simulink model "FourRigidBar3D"  (R2025b)
settings: Solver=VariableStepAuto  StartTime=0.0  StopTime=10.0  RelTol=1e-3
undefined symbols (not defined in the file): I2_G, I4_G, InvDyn, l2, l4, m2, m4, pass, sig4, ureal, uss
libraries: RCTblocks x138
(part 1 of 2)
settings Model: Creator=d.alazard  LastModifiedBy=andre
settings SolverCC: AlgebraicLoopSolver=TrustRegion
settings DebuggingCC: AlgebraicLoopMsg=none  UnconnectedInputMsg=warning  UnconnectedOutputMsg=warning  UnconnectedLineMsg=warning
settings ModelReferenceCC: EnableRefExpFcnMdlSchedulingChecks=on
settings RTWCC: GPUComputeCapability=3.5  DLArmComputeVersion=19.05

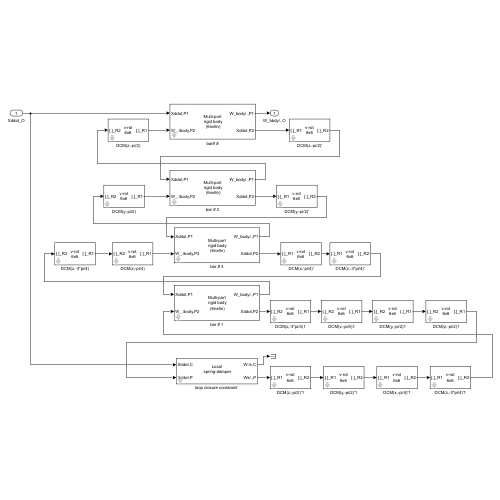
[thumbnail: Simulink's stored preview of the top-level diagram]
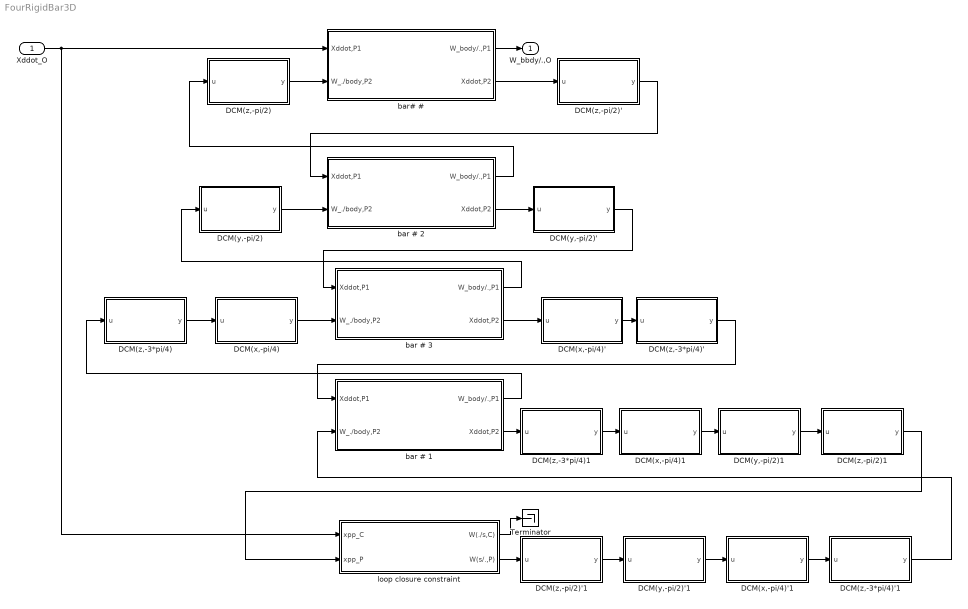
== system FourRigidBar3D ==
  Xddot_O : Inport
  DCM(x,-pi/4) : Subsystem  mask(6x6 rotation matrix (around a given axis)){ra=[1;0;0], theta=-pi/4, transp=off}
      mask prompts: ra "Rotation axis (3x1 vector)"; theta "Angle (rad)"; transp "Matrix transposed"
      mask help:
      | For 6 d.o.f. body motion (3 translations and 3 rotations), this block Implement the 6x6 rotation matrix (or its transposed) for a given angle around a given axis.
      |
      | Angle  (rad) can be an uncertain parameter declared with "ureal" with mode 'Range'
      | Ex: ureal('NAME',0,'Range',[-pi pi])
      | Then, ULINEARIZE will provide a model involving the block named "tan_NAME_div4".
      mask init:
      | vUrotation3x3
      mask Help: web('Doc6vurotation.html','-browser')
      mask Display:
      | disp('v-rot\n6x6')
      | if transp
      |     port_label('input', 1, '[.]_R1')
      |     port_label('output', 1, '[.]_R2')
      | else
      |     port_label('input', 1, '[.]_R2')
      |     port_label('output', 1, '[.]_R1')
      | end
  DCM(x,-pi/4)' : Subsystem  mask(6x6 rotation matrix (around a given axis)){ra=[1;0;0], theta=-pi/4, transp=on}
      mask prompts: ra "Rotation axis (3x1 vector)"; theta "Angle (rad)"; transp "Matrix transposed"
      mask help:
      | For 6 d.o.f. body motion (3 translations and 3 rotations), this block Implement the 6x6 rotation matrix (or its transposed) for a given angle around a given axis.
      |
      | Angle  (rad) can be an uncertain parameter declared with "ureal" with mode 'Range'
      | Ex: ureal('NAME',0,'Range',[-pi pi])
      | Then, ULINEARIZE will provide a model involving the block named "tan_NAME_div4".
      mask init:
      | vUrotation3x3
      mask Help: web('Doc6vurotation.html','-browser')
      mask Display:
      | disp('v-rot\n6x6')
      | if transp
      |     port_label('input', 1, '[.]_R1')
      |     port_label('output', 1, '[.]_R2')
      | else
      |     port_label('input', 1, '[.]_R2')
      |     port_label('output', 1, '[.]_R1')
      | end
  DCM(x,-pi/4)'1 : Subsystem  mask(6x6 rotation matrix (around a given axis)){ra=[1;0;0], theta=-pi/4, transp=on}
      mask prompts: ra "Rotation axis (3x1 vector)"; theta "Angle (rad)"; transp "Matrix transposed"
      mask help:
      | For 6 d.o.f. body motion (3 translations and 3 rotations), this block Implement the 6x6 rotation matrix (or its transposed) for a given angle around a given axis.
      |
      | Angle  (rad) can be an uncertain parameter declared with "ureal" with mode 'Range'
      | Ex: ureal('NAME',0,'Range',[-pi pi])
      | Then, ULINEARIZE will provide a model involving the block named "tan_NAME_div4".
      mask init:
      | vUrotation3x3
      mask Help: web('Doc6vurotation.html','-browser')
      mask Display:
      | disp('v-rot\n6x6')
      | if transp
      |     port_label('input', 1, '[.]_R1')
      |     port_label('output', 1, '[.]_R2')
      | else
      |     port_label('input', 1, '[.]_R2')
      |     port_label('output', 1, '[.]_R1')
      | end
  DCM(x,-pi/4)1 : Subsystem  mask(6x6 rotation matrix (around a given axis)){ra=[1;0;0], theta=-pi/4, transp=off}
      mask prompts: ra "Rotation axis (3x1 vector)"; theta "Angle (rad)"; transp "Matrix transposed"
      mask help:
      | For 6 d.o.f. body motion (3 translations and 3 rotations), this block Implement the 6x6 rotation matrix (or its transposed) for a given angle around a given axis.
      |
      | Angle  (rad) can be an uncertain parameter declared with "ureal" with mode 'Range'
      | Ex: ureal('NAME',0,'Range',[-pi pi])
      | Then, ULINEARIZE will provide a model involving the block named "tan_NAME_div4".
      mask init:
      | vUrotation3x3
      mask Help: web('Doc6vurotation.html','-browser')
      mask Display:
      | disp('v-rot\n6x6')
      | if transp
      |     port_label('input', 1, '[.]_R1')
      |     port_label('output', 1, '[.]_R2')
      | else
      |     port_label('input', 1, '[.]_R2')
      |     port_label('output', 1, '[.]_R1')
      | end
  DCM(y,-pi/2) : Subsystem  mask(6x6 rotation matrix (around a given axis)){ra=[0;1;0], theta=-pi/2, transp=off}
      mask prompts: ra "Rotation axis (3x1 vector)"; theta "Angle (rad)"; transp "Matrix transposed"
      mask help:
      | For 6 d.o.f. body motion (3 translations and 3 rotations), this block Implement the 6x6 rotation matrix (or its transposed) for a given angle around a given axis.
      |
      | Angle  (rad) can be an uncertain parameter declared with "ureal" with mode 'Range'
      | Ex: ureal('NAME',0,'Range',[-pi pi])
      | Then, ULINEARIZE will provide a model involving the block named "tan_NAME_div4".
      mask init:
      | vUrotation3x3
      mask Help: web('Doc6vurotation.html','-browser')
      mask Display:
      | disp('v-rot\n6x6')
      | if transp
      |     port_label('input', 1, '[.]_R1')
      |     port_label('output', 1, '[.]_R2')
      | else
      |     port_label('input', 1, '[.]_R2')
      |     port_label('output', 1, '[.]_R1')
      | end
  DCM(y,-pi/2)' : Subsystem  mask(6x6 rotation matrix (around a given axis)){ra=[0;1;0], theta=-pi/2, transp=on}
      mask prompts: ra "Rotation axis (3x1 vector)"; theta "Angle (rad)"; transp "Matrix transposed"
      mask help:
      | For 6 d.o.f. body motion (3 translations and 3 rotations), this block Implement the 6x6 rotation matrix (or its transposed) for a given angle around a given axis.
      |
      | Angle  (rad) can be an uncertain parameter declared with "ureal" with mode 'Range'
      | Ex: ureal('NAME',0,'Range',[-pi pi])
      | Then, ULINEARIZE will provide a model involving the block named "tan_NAME_div4".
      mask init:
      | vUrotation3x3
      mask Help: web('Doc6vurotation.html','-browser')
      mask Display:
      | disp('v-rot\n6x6')
      | if transp
      |     port_label('input', 1, '[.]_R1')
      |     port_label('output', 1, '[.]_R2')
      | else
      |     port_label('input', 1, '[.]_R2')
      |     port_label('output', 1, '[.]_R1')
      | end
  DCM(y,-pi/2)'1 : Subsystem  mask(6x6 rotation matrix (around a given axis)){ra=[0;1;0], theta=-pi/2, transp=on}
      mask prompts: ra "Rotation axis (3x1 vector)"; theta "Angle (rad)"; transp "Matrix transposed"
      mask help:
      | For 6 d.o.f. body motion (3 translations and 3 rotations), this block Implement the 6x6 rotation matrix (or its transposed) for a given angle around a given axis.
      |
      | Angle  (rad) can be an uncertain parameter declared with "ureal" with mode 'Range'
      | Ex: ureal('NAME',0,'Range',[-pi pi])
      | Then, ULINEARIZE will provide a model involving the block named "tan_NAME_div4".
      mask init:
      | vUrotation3x3
      mask Help: web('Doc6vurotation.html','-browser')
      mask Display:
      | disp('v-rot\n6x6')
      | if transp
      |     port_label('input', 1, '[.]_R1')
      |     port_label('output', 1, '[.]_R2')
      | else
      |     port_label('input', 1, '[.]_R2')
      |     port_label('output', 1, '[.]_R1')
      | end
  DCM(y,-pi/2)1 : Subsystem  mask(6x6 rotation matrix (around a given axis)){ra=[0;1;0], theta=-pi/2, transp=off}
      mask prompts: ra "Rotation axis (3x1 vector)"; theta "Angle (rad)"; transp "Matrix transposed"
      mask help:
      | For 6 d.o.f. body motion (3 translations and 3 rotations), this block Implement the 6x6 rotation matrix (or its transposed) for a given angle around a given axis.
      |
      | Angle  (rad) can be an uncertain parameter declared with "ureal" with mode 'Range'
      | Ex: ureal('NAME',0,'Range',[-pi pi])
      | Then, ULINEARIZE will provide a model involving the block named "tan_NAME_div4".
      mask init:
      | vUrotation3x3
      mask Help: web('Doc6vurotation.html','-browser')
      mask Display:
      | disp('v-rot\n6x6')
      | if transp
      |     port_label('input', 1, '[.]_R1')
      |     port_label('output', 1, '[.]_R2')
      | else
      |     port_label('input', 1, '[.]_R2')
      |     port_label('output', 1, '[.]_R1')
      | end
  DCM(z,-3*pi/4) : Subsystem  mask(6x6 rotation matrix (around a given axis)){ra=[0;0;1], theta=-3*pi/4, transp=off}
      mask prompts: ra "Rotation axis (3x1 vector)"; theta "Angle (rad)"; transp "Matrix transposed"
      mask help:
      | For 6 d.o.f. body motion (3 translations and 3 rotations), this block Implement the 6x6 rotation matrix (or its transposed) for a given angle around a given axis.
      |
      | Angle  (rad) can be an uncertain parameter declared with "ureal" with mode 'Range'
      | Ex: ureal('NAME',0,'Range',[-pi pi])
      | Then, ULINEARIZE will provide a model involving the block named "tan_NAME_div4".
      mask init:
      | vUrotation3x3
      mask Help: web('Doc6vurotation.html','-browser')
      mask Display:
      | disp('v-rot\n6x6')
      | if transp
      |     port_label('input', 1, '[.]_R1')
      |     port_label('output', 1, '[.]_R2')
      | else
      |     port_label('input', 1, '[.]_R2')
      |     port_label('output', 1, '[.]_R1')
      | end
  DCM(z,-3*pi/4)' : Subsystem  mask(6x6 rotation matrix (around a given axis)){ra=[0;0;1], theta=-3*pi/4, transp=on}
      mask prompts: ra "Rotation axis (3x1 vector)"; theta "Angle (rad)"; transp "Matrix transposed"
      mask help:
      | For 6 d.o.f. body motion (3 translations and 3 rotations), this block Implement the 6x6 rotation matrix (or its transposed) for a given angle around a given axis.
      |
      | Angle  (rad) can be an uncertain parameter declared with "ureal" with mode 'Range'
      | Ex: ureal('NAME',0,'Range',[-pi pi])
      | Then, ULINEARIZE will provide a model involving the block named "tan_NAME_div4".
      mask init:
      | vUrotation3x3
      mask Help: web('Doc6vurotation.html','-browser')
      mask Display:
      | disp('v-rot\n6x6')
      | if transp
      |     port_label('input', 1, '[.]_R1')
      |     port_label('output', 1, '[.]_R2')
      | else
      |     port_label('input', 1, '[.]_R2')
      |     port_label('output', 1, '[.]_R1')
      | end
  DCM(z,-3*pi/4)'1 : Subsystem  mask(6x6 rotation matrix (around a given axis)){ra=[0;0;1], theta=-3*pi/4, transp=on}
      mask prompts: ra "Rotation axis (3x1 vector)"; theta "Angle (rad)"; transp "Matrix transposed"
      mask help:
      | For 6 d.o.f. body motion (3 translations and 3 rotations), this block Implement the 6x6 rotation matrix (or its transposed) for a given angle around a given axis.
      |
      | Angle  (rad) can be an uncertain parameter declared with "ureal" with mode 'Range'
      | Ex: ureal('NAME',0,'Range',[-pi pi])
      | Then, ULINEARIZE will provide a model involving the block named "tan_NAME_div4".
      mask init:
      | vUrotation3x3
      mask Help: web('Doc6vurotation.html','-browser')
      mask Display:
      | disp('v-rot\n6x6')
      | if transp
      |     port_label('input', 1, '[.]_R1')
      |     port_label('output', 1, '[.]_R2')
      | else
      |     port_label('input', 1, '[.]_R2')
      |     port_label('output', 1, '[.]_R1')
      | end
  DCM(z,-3*pi/4)1 : Subsystem  mask(6x6 rotation matrix (around a given axis)){ra=[0;0;1], theta=-3*pi/4, transp=off}
      mask prompts: ra "Rotation axis (3x1 vector)"; theta "Angle (rad)"; transp "Matrix transposed"
      mask help:
      | For 6 d.o.f. body motion (3 translations and 3 rotations), this block Implement the 6x6 rotation matrix (or its transposed) for a given angle around a given axis.
      |
      | Angle  (rad) can be an uncertain parameter declared with "ureal" with mode 'Range'
      | Ex: ureal('NAME',0,'Range',[-pi pi])
      | Then, ULINEARIZE will provide a model involving the block named "tan_NAME_div4".
      mask init:
      | vUrotation3x3
      mask Help: web('Doc6vurotation.html','-browser')
      mask Display:
      | disp('v-rot\n6x6')
      | if transp
      |     port_label('input', 1, '[.]_R1')
      |     port_label('output', 1, '[.]_R2')
      | else
      |     port_label('input', 1, '[.]_R2')
      |     port_label('output', 1, '[.]_R1')
      | end
  DCM(z,-pi/2) : Subsystem  mask(6x6 rotation matrix (around a given axis)){ra=[0;0;1], theta=-pi/2, transp=off}
      mask prompts: ra "Rotation axis (3x1 vector)"; theta "Angle (rad)"; transp "Matrix transposed"
      mask help:
      | For 6 d.o.f. body motion (3 translations and 3 rotations), this block Implement the 6x6 rotation matrix (or its transposed) for a given angle around a given axis.
      |
      | Angle  (rad) can be an uncertain parameter declared with "ureal" with mode 'Range'
      | Ex: ureal('NAME',0,'Range',[-pi pi])
      | Then, ULINEARIZE will provide a model involving the block named "tan_NAME_div4".
      mask init:
      | vUrotation3x3
      mask Help: web('Doc6vurotation.html','-browser')
      mask Display:
      | disp('v-rot\n6x6')
      | if transp
      |     port_label('input', 1, '[.]_R1')
      |     port_label('output', 1, '[.]_R2')
      | else
      |     port_label('input', 1, '[.]_R2')
      |     port_label('output', 1, '[.]_R1')
      | end
  DCM(z,-pi/2)' : Subsystem  mask(6x6 rotation matrix (around a given axis)){ra=[0;0;1], theta=-pi/2, transp=on}
      mask prompts: ra "Rotation axis (3x1 vector)"; theta "Angle (rad)"; transp "Matrix transposed"
      mask help:
      | For 6 d.o.f. body motion (3 translations and 3 rotations), this block Implement the 6x6 rotation matrix (or its transposed) for a given angle around a given axis.
      |
      | Angle  (rad) can be an uncertain parameter declared with "ureal" with mode 'Range'
      | Ex: ureal('NAME',0,'Range',[-pi pi])
      | Then, ULINEARIZE will provide a model involving the block named "tan_NAME_div4".
      mask init:
      | vUrotation3x3
      mask Help: web('Doc6vurotation.html','-browser')
      mask Display:
      | disp('v-rot\n6x6')
      | if transp
      |     port_label('input', 1, '[.]_R1')
      |     port_label('output', 1, '[.]_R2')
      | else
      |     port_label('input', 1, '[.]_R2')
      |     port_label('output', 1, '[.]_R1')
      | end
  DCM(z,-pi/2)'1 : Subsystem  mask(6x6 rotation matrix (around a given axis)){ra=[0;0;1], theta=-pi/2, transp=on}
      mask prompts: ra "Rotation axis (3x1 vector)"; theta "Angle (rad)"; transp "Matrix transposed"
      mask help:
      | For 6 d.o.f. body motion (3 translations and 3 rotations), this block Implement the 6x6 rotation matrix (or its transposed) for a given angle around a given axis.
      |
      | Angle  (rad) can be an uncertain parameter declared with "ureal" with mode 'Range'
      | Ex: ureal('NAME',0,'Range',[-pi pi])
      | Then, ULINEARIZE will provide a model involving the block named "tan_NAME_div4".
      mask init:
      | vUrotation3x3
      mask Help: web('Doc6vurotation.html','-browser')
      mask Display:
      | disp('v-rot\n6x6')
      | if transp
      |     port_label('input', 1, '[.]_R1')
      |     port_label('output', 1, '[.]_R2')
      | else
      |     port_label('input', 1, '[.]_R2')
      |     port_label('output', 1, '[.]_R1')
      | end
  DCM(z,-pi/2)1 : Subsystem  mask(6x6 rotation matrix (around a given axis)){ra=[0;0;1], theta=-pi/2, transp=off}
      mask prompts: ra "Rotation axis (3x1 vector)"; theta "Angle (rad)"; transp "Matrix transposed"
      mask help:
      | For 6 d.o.f. body motion (3 translations and 3 rotations), this block Implement the 6x6 rotation matrix (or its transposed) for a given angle around a given axis.
      |
      | Angle  (rad) can be an uncertain parameter declared with "ureal" with mode 'Range'
      | Ex: ureal('NAME',0,'Range',[-pi pi])
      | Then, ULINEARIZE will provide a model involving the block named "tan_NAME_div4".
      mask init:
      | vUrotation3x3
      mask Help: web('Doc6vurotation.html','-browser')
      mask Display:
      | disp('v-rot\n6x6')
      | if transp
      |     port_label('input', 1, '[.]_R1')
      |     port_label('output', 1, '[.]_R2')
      | else
      |     port_label('input', 1, '[.]_R2')
      |     port_label('output', 1, '[.]_R1')
      | end
  Terminator : Terminator
  bar # 1 : Subsystem  mask(Multi-port rigid body (6nx6n)){m=m4, Ig=I4_G, OG=[l4/2;0;0], n=2, numinv=1, OP1=[0;0;0], OP2=[l4;0;0], OP3=[ureal('P3_y',1,'percent',10);0;0], OP4=[0;0;0], OP5=[0;0;0]}
      mask prompts: m "Mass (Kg)"; Ig "Inertia (at G, Kg m^2)"; OG "OG (3x1 vector, m)"; n "Number of ports"; numinv "Port to be inverted"; OP1 "OP1 (3x1 vector, m)"; OP2 "OP2 (3x1 vector, m)"; OP3 "OP3 (3x1 vector, m)"; OP4 "OP4 (3x1 vector, m)"; OP5 "OP5 (3x1 vector,m)"
      mask help:
      | 6nx6n dynamic model of a rigid body at n given points (ports) between wrenches applied at the n points (input) and acceleration twists at these points (output).
      |
      | 0: the reference point
      | G: the center of mass
      | Pi (i=1:n): the n given connection points (n<6).
      |
      | All parameters are expressed in the body frame.
      | Each parameter can be an uncertain parameter declared with "ureal"
      |
      | The 6x6 channel associated to one port can be inverted: then the input of this channel is the acceleration twist imposed at this point and the output is the wrench applied by this body.
      mask init:
      | MultiPortRigidBody
      mask Help: web('Docmultiportrigidbody.html','-browser')
      mask TypeOptions n: 1 | 2 | 3 | 4 | 5
      mask TypeOptions numinv: none | 1 | 2 | 3 | 4 | 5
      mask DialogControl ParameterGroupVar Prompt: Main parameters
      mask DialogControl port1 Prompt: Port #1
      mask DialogControl port2 Prompt: #2
      mask DialogControl port3 Prompt: #3
      mask DialogControl port4 Prompt: #4
      mask DialogControl port5 Prompt: #5
      mask Display:
      | disp('Multi-port\n rigid body\n (6nx6n)')
      | if n==1,
      |     if numinv-1==1,
      |         port_label('input', 1,'Xddot,P')
      |         port_label('output',1,'W_body/.,P')
      |     else
      |         port_label('input', 1,'W_./body,P')
      |         port_label('output',1,'Xddot,P')
      |     end
      | else
      |     for ii=1:n
      |         if numinv==ii+1,
      |             port_label('output',ii,['W_body/.,P',num2str(ii)])
      |             port_label('input', ii,['Xddot,P',num2str(ii)])
      |         else
      |             port_label('input', ii,['W_./body,P',num2str(ii)])
      |             port_label('output',ii,['Xddot,P',num2str(ii)])
      |         end
      |     end
      | end
  bar # 2 : Subsystem  mask(Multi-port rigid body (6nx6n)){m=m2, Ig=I2_G, OG=[l2/2;0;0], n=2, numinv=1, OP1=[0;0;0], OP2=[l2;0;0], OP3=[ureal('P3_y',1,'percent',10);0;0], OP4=[0;0;0], OP5=[0;0;0]}
      mask prompts: m "Mass (Kg)"; Ig "Inertia (at G, Kg m^2)"; OG "OG (3x1 vector, m)"; n "Number of ports"; numinv "Port to be inverted"; OP1 "OP1 (3x1 vector, m)"; OP2 "OP2 (3x1 vector, m)"; OP3 "OP3 (3x1 vector, m)"; OP4 "OP4 (3x1 vector, m)"; OP5 "OP5 (3x1 vector,m)"
      mask help:
      | 6nx6n dynamic model of a rigid body at n given points (ports) between wrenches applied at the n points (input) and acceleration twists at these points (output).
      |
      | 0: the reference point
      | G: the center of mass
      | Pi (i=1:n): the n given connection points (n<6).
      |
      | All parameters are expressed in the body frame.
      | Each parameter can be an uncertain parameter declared with "ureal"
      |
      | The 6x6 channel associated to one port can be inverted: then the input of this channel is the acceleration twist imposed at this point and the output is the wrench applied by this body.
      mask init:
      | MultiPortRigidBody
      mask Help: web('Docmultiportrigidbody.html','-browser')
      mask TypeOptions n: 1 | 2 | 3 | 4 | 5
      mask TypeOptions numinv: none | 1 | 2 | 3 | 4 | 5
      mask DialogControl ParameterGroupVar Prompt: Main parameters
      mask DialogControl port1 Prompt: Port #1
      mask DialogControl port2 Prompt: #2
      mask DialogControl port3 Prompt: #3
      mask DialogControl port4 Prompt: #4
      mask DialogControl port5 Prompt: #5
      mask Display:
      | disp('Multi-port\n rigid body\n (6nx6n)')
      | if n==1,
      |     if numinv-1==1,
      |         port_label('input', 1,'Xddot,P')
      |         port_label('output',1,'W_body/.,P')
      |     else
      |         port_label('input', 1,'W_./body,P')
      |         port_label('output',1,'Xddot,P')
      |     end
      | else
      |     for ii=1:n
      |         if numinv==ii+1,
      |             port_label('output',ii,['W_body/.,P',num2str(ii)])
      |             port_label('input', ii,['Xddot,P',num2str(ii)])
      |         else
      |             port_label('input', ii,['W_./body,P',num2str(ii)])
      |             port_label('output',ii,['Xddot,P',num2str(ii)])
      |         end
      |     end
      | end
  bar # 3 : Subsystem  mask(Multi-port rigid body (6nx6n)){m=m2, Ig=I2_G, OG=[l2/2;0;0], n=2, numinv=1, OP1=[0;0;0], OP2=[l2;0;0], OP3=[ureal('P3_y',1,'percent',10);0;0], OP4=[0;0;0], OP5=[0;0;0]}
      mask prompts: m "Mass (Kg)"; Ig "Inertia (at G, Kg m^2)"; OG "OG (3x1 vector, m)"; n "Number of ports"; numinv "Port to be inverted"; OP1 "OP1 (3x1 vector, m)"; OP2 "OP2 (3x1 vector, m)"; OP3 "OP3 (3x1 vector, m)"; OP4 "OP4 (3x1 vector, m)"; OP5 "OP5 (3x1 vector,m)"
      mask help:
      | 6nx6n dynamic model of a rigid body at n given points (ports) between wrenches applied at the n points (input) and acceleration twists at these points (output).
      |
      | 0: the reference point
      | G: the center of mass
      | Pi (i=1:n): the n given connection points (n<6).
      |
      | All parameters are expressed in the body frame.
      | Each parameter can be an uncertain parameter declared with "ureal"
      |
      | The 6x6 channel associated to one port can be inverted: then the input of this channel is the acceleration twist imposed at this point and the output is the wrench applied by this body.
      mask init:
      | MultiPortRigidBody
      mask Help: web('Docmultiportrigidbody.html','-browser')
      mask TypeOptions n: 1 | 2 | 3 | 4 | 5
      mask TypeOptions numinv: none | 1 | 2 | 3 | 4 | 5
      mask DialogControl ParameterGroupVar Prompt: Main parameters
      mask DialogControl port1 Prompt: Port #1
      mask DialogControl port2 Prompt: #2
      mask DialogControl port3 Prompt: #3
      mask DialogControl port4 Prompt: #4
      mask DialogControl port5 Prompt: #5
      mask Display:
      | disp('Multi-port\n rigid body\n (6nx6n)')
      | if n==1,
      |     if numinv-1==1,
      |         port_label('input', 1,'Xddot,P')
      |         port_label('output',1,'W_body/.,P')
      |     else
      |         port_label('input', 1,'W_./body,P')
      |         port_label('output',1,'Xddot,P')
      |     end
      | else
      |     for ii=1:n
      |         if numinv==ii+1,
      |             port_label('output',ii,['W_body/.,P',num2str(ii)])
      |             port_label('input', ii,['Xddot,P',num2str(ii)])
      |         else
      |             port_label('input', ii,['W_./body,P',num2str(ii)])
      |             port_label('output',ii,['Xddot,P',num2str(ii)])
      |         end
      |     end
      | end
  bar# # : Subsystem  mask(Multi-port rigid body (6nx6n)){m=m2, Ig=I2_G, OG=[l2/2;0;0], n=2, numinv=1, OP1=[0;0;0], OP2=[l2;0;0], OP3=[ureal('P3_y',1,'percent',10);0;0], OP4=[0;0;0], OP5=[0;0;0]}
      mask prompts: m "Mass (Kg)"; Ig "Inertia (at G, Kg m^2)"; OG "OG (3x1 vector, m)"; n "Number of ports"; numinv "Port to be inverted"; OP1 "OP1 (3x1 vector, m)"; OP2 "OP2 (3x1 vector, m)"; OP3 "OP3 (3x1 vector, m)"; OP4 "OP4 (3x1 vector, m)"; OP5 "OP5 (3x1 vector,m)"
      mask help:
      | 6nx6n dynamic model of a rigid body at n given points (ports) between wrenches applied at the n points (input) and acceleration twists at these points (output).
      |
      | 0: the reference point
      | G: the center of mass
      | Pi (i=1:n): the n given connection points (n<6).
      |
      | All parameters are expressed in the body frame.
      | Each parameter can be an uncertain parameter declared with "ureal"
      |
      | The 6x6 channel associated to one port can be inverted: then the input of this channel is the acceleration twist imposed at this point and the output is the wrench applied by this body.
      mask init:
      | MultiPortRigidBody
      mask Help: web('Docmultiportrigidbody.html','-browser')
      mask TypeOptions n: 1 | 2 | 3 | 4 | 5
      mask TypeOptions numinv: none | 1 | 2 | 3 | 4 | 5
      mask DialogControl ParameterGroupVar Prompt: Main parameters
      mask DialogControl port1 Prompt: Port #1
      mask DialogControl port2 Prompt: #2
      mask DialogControl port3 Prompt: #3
      mask DialogControl port4 Prompt: #4
      mask DialogControl port5 Prompt: #5
      mask Display:
      | disp('Multi-port\n rigid body\n (6nx6n)')
      | if n==1,
      |     if numinv-1==1,
      |         port_label('input', 1,'Xddot,P')
      |         port_label('output',1,'W_body/.,P')
      |     else
      |         port_label('input', 1,'W_./body,P')
      |         port_label('output',1,'Xddot,P')
      |     end
      | else
      |     for ii=1:n
      |         if numinv==ii+1,
      |             port_label('output',ii,['W_body/.,P',num2str(ii)])
      |             port_label('input', ii,['Xddot,P',num2str(ii)])
      |         else
      |             port_label('input', ii,['W_./body,P',num2str(ii)])
      |             port_label('output',ii,['Xddot,P',num2str(ii)])
      |         end
      |     end
      | end
  "loop closure constraint " : Subsystem  mask(Local stiffness damper){K_O=diag([1 1 1 2 2 2]), D_O=diag([10 10 10 20 20 20]), OP=[0;0;0], OC=[0;0;0]}
      mask prompts: K_O "6x6 stiffness matrix at point O (N/m, Nm/rad)"; D_O "6x6 damping matrix  at point O (Ns/m, Nms/rad)"; OP "OP (3x1 vector (m)"; OC "OC (3x1 vector  (m)"
      mask help:
      | 12x12 TITOP model of a massless spring-damper system between:
      |   * the 2 acceleration twists (inputs)  at the parent port (point P) and the child port (point C).
      |   *  the outside wrench applied to the spring-damper  at point C and the wrench by the spring-damper to outside at point P.
      | The model is expressed In the inherit reference frame.
      |
      | All the parameters can be declared as uncertain parameters (ureal(...)).
      mask init:
      | TAU_OC=kinematic_model([0;0;0],OC);
      | TAU_OP=kinematic_model([0;0;0],OP);
      mask Help: web('Doc_6DOFs_spring_damper.html','-browser')
      mask DialogControl ParameterGroupVar Prompt: Main parameters
      mask Display:
      | disp('Local\n spring-damper\n')
      | 
      | port_label('input', 1,'Xddot,C')
      | port_label('output',1,'W./s,C')
      | port_label('input', 2,'Xddot,P')
      | port_label('output',2,'Ws/.,P')
  W_bbdy/.,O : Outport
  wires:
  Xddot_O/1 -> "loop closure constraint "/1(xpp_C), bar# #/1(Xddot,P1)
  bar# #/2(Xddot,P2) -> DCM(z,-pi/2)'/1(u)
  DCM(z,-pi/2)/1(y) -> bar# #/2(W_./body,P2)
  DCM(z,-pi/2)'/1(y) -> bar # 2/1(Xddot,P1)
  bar # 2/1(W_body/.,P1) -> DCM(z,-pi/2)/1(u)
  bar # 2/2(Xddot,P2) -> DCM(y,-pi/2)'/1(u)
  DCM(y,-pi/2)/1(y) -> bar # 2/2(W_./body,P2)
  DCM(y,-pi/2)'/1(y) -> bar # 3/1(Xddot,P1)
  bar # 3/1(W_body/.,P1) -> DCM(y,-pi/2)/1(u)
  bar # 3/2(Xddot,P2) -> DCM(x,-pi/4)'/1(u)
  DCM(x,-pi/4)/1(y) -> bar # 3/2(W_./body,P2)
  DCM(x,-pi/4)'/1(y) -> DCM(z,-3*pi/4)'/1(u)
  DCM(z,-3*pi/4)/1(y) -> DCM(x,-pi/4)/1(u)
  DCM(z,-3*pi/4)'/1(y) -> bar # 1/1(Xddot,P1)
  bar # 1/1(W_body/.,P1) -> DCM(z,-3*pi/4)/1(u)
  bar # 1/2(Xddot,P2) -> DCM(z,-3*pi/4)1/1(u)
  DCM(z,-3*pi/4)1/1(y) -> DCM(x,-pi/4)1/1(u)
  DCM(x,-pi/4)1/1(y) -> DCM(y,-pi/2)1/1(u)
  DCM(y,-pi/2)1/1(y) -> DCM(z,-pi/2)1/1(u)
  DCM(z,-pi/2)1/1(y) -> "loop closure constraint "/2(xpp_P)
  "loop closure constraint "/2(W(s/.,P)) -> DCM(z,-pi/2)'1/1(u)
  bar# #/1(W_body/.,P1) -> W_bbdy/.,O/1
  DCM(z,-pi/2)'1/1(y) -> DCM(y,-pi/2)'1/1(u)
  DCM(y,-pi/2)'1/1(y) -> DCM(x,-pi/4)'1/1(u)
  DCM(x,-pi/4)'1/1(y) -> DCM(z,-3*pi/4)'1/1(u)
  DCM(z,-3*pi/4)'1/1(y) -> bar # 1/2(W_./body,P2)
  "loop closure constraint "/1(W(./s,C)) -> Terminator/1

== system FourRigidBar3D/DCM(x,-pi//4) ==
  u : Inport  PortDimensions=6
  Demux : Demux  Outputs=[3 3]
  Mux : Mux  Inputs=[3 3]
  Subsystem : Subsystem
  Subsystem1 : Subsystem
  y : Outport  VectorParamsAs1DForOutWhenUnconnected=off
  wires:
  Subsystem1/1(Out1) -> Mux/2
  Subsystem/1(Out1) -> Mux/1
  Demux/2 -> Subsystem1/1(In1)
  Demux/1 -> Subsystem/1(In1)
  u/1 -> Demux/1
  Mux/1 -> y/1

== system FourRigidBar3D/DCM(x,-pi//4)' ==
  u : Inport  PortDimensions=6
  Demux : Demux  Outputs=[3 3]
  Mux : Mux  Inputs=[3 3]
  Subsystem : Subsystem
  Subsystem1 : Subsystem
  y : Outport  VectorParamsAs1DForOutWhenUnconnected=off
  wires:
  Subsystem1/1(Out1) -> Mux/2
  Subsystem/1(Out1) -> Mux/1
  Demux/2 -> Subsystem1/1(In1)
  Demux/1 -> Subsystem/1(In1)
  u/1 -> Demux/1
  Mux/1 -> y/1

== system FourRigidBar3D/DCM(x,-pi//4)'1 ==
  u : Inport  PortDimensions=6
  Demux : Demux  Outputs=[3 3]
  Mux : Mux  Inputs=[3 3]
  Subsystem : Subsystem
  Subsystem1 : Subsystem
  y : Outport  VectorParamsAs1DForOutWhenUnconnected=off
  wires:
  Subsystem1/1(Out1) -> Mux/2
  Subsystem/1(Out1) -> Mux/1
  Demux/2 -> Subsystem1/1(In1)
  Demux/1 -> Subsystem/1(In1)
  u/1 -> Demux/1
  Mux/1 -> y/1

== system FourRigidBar3D/DCM(x,-pi//4)1 ==
  u : Inport  PortDimensions=6
  Demux : Demux  Outputs=[3 3]
  Mux : Mux  Inputs=[3 3]
  Subsystem : Subsystem
  Subsystem1 : Subsystem
  y : Outport  VectorParamsAs1DForOutWhenUnconnected=off
  wires:
  Subsystem1/1(Out1) -> Mux/2
  Subsystem/1(Out1) -> Mux/1
  Demux/2 -> Subsystem1/1(In1)
  Demux/1 -> Subsystem/1(In1)
  u/1 -> Demux/1
  Mux/1 -> y/1

== system FourRigidBar3D/DCM(y,-pi//2) ==
  u : Inport  PortDimensions=6
  Demux : Demux  Outputs=[3 3]
  Mux : Mux  Inputs=[3 3]
  Subsystem : Subsystem
  Subsystem1 : Subsystem
  y : Outport  VectorParamsAs1DForOutWhenUnconnected=off
  wires:
  Subsystem1/1(Out1) -> Mux/2
  Subsystem/1(Out1) -> Mux/1
  Demux/2 -> Subsystem1/1(In1)
  Demux/1 -> Subsystem/1(In1)
  u/1 -> Demux/1
  Mux/1 -> y/1

== system FourRigidBar3D/DCM(y,-pi//2)' ==
  u : Inport  PortDimensions=6
  Demux : Demux  Outputs=[3 3]
  Mux : Mux  Inputs=[3 3]
  Subsystem : Subsystem
  Subsystem1 : Subsystem
  y : Outport  VectorParamsAs1DForOutWhenUnconnected=off
  wires:
  Subsystem1/1(Out1) -> Mux/2
  Subsystem/1(Out1) -> Mux/1
  Demux/2 -> Subsystem1/1(In1)
  Demux/1 -> Subsystem/1(In1)
  u/1 -> Demux/1
  Mux/1 -> y/1

== system FourRigidBar3D/DCM(y,-pi//2)'1 ==
  u : Inport  PortDimensions=6
  Demux : Demux  Outputs=[3 3]
  Mux : Mux  Inputs=[3 3]
  Subsystem : Subsystem
  Subsystem1 : Subsystem
  y : Outport  VectorParamsAs1DForOutWhenUnconnected=off
  wires:
  Subsystem1/1(Out1) -> Mux/2
  Subsystem/1(Out1) -> Mux/1
  Demux/2 -> Subsystem1/1(In1)
  Demux/1 -> Subsystem/1(In1)
  u/1 -> Demux/1
  Mux/1 -> y/1

== system FourRigidBar3D/DCM(y,-pi//2)1 ==
  u : Inport  PortDimensions=6
  Demux : Demux  Outputs=[3 3]
  Mux : Mux  Inputs=[3 3]
  Subsystem : Subsystem
  Subsystem1 : Subsystem
  y : Outport  VectorParamsAs1DForOutWhenUnconnected=off
  wires:
  Subsystem1/1(Out1) -> Mux/2
  Subsystem/1(Out1) -> Mux/1
  Demux/2 -> Subsystem1/1(In1)
  Demux/1 -> Subsystem/1(In1)
  u/1 -> Demux/1
  Mux/1 -> y/1

== system FourRigidBar3D/DCM(z,-3*pi//4) ==
  u : Inport  PortDimensions=6
  Demux : Demux  Outputs=[3 3]
  Mux : Mux  Inputs=[3 3]
  Subsystem : Subsystem
  Subsystem1 : Subsystem
  y : Outport  VectorParamsAs1DForOutWhenUnconnected=off
  wires:
  Subsystem1/1(Out1) -> Mux/2
  Subsystem/1(Out1) -> Mux/1
  Demux/2 -> Subsystem1/1(In1)
  Demux/1 -> Subsystem/1(In1)
  u/1 -> Demux/1
  Mux/1 -> y/1

== system FourRigidBar3D/DCM(z,-3*pi//4)' ==
  u : Inport  PortDimensions=6
  Demux : Demux  Outputs=[3 3]
  Mux : Mux  Inputs=[3 3]
  Subsystem : Subsystem
  Subsystem1 : Subsystem
  y : Outport  VectorParamsAs1DForOutWhenUnconnected=off
  wires:
  Subsystem1/1(Out1) -> Mux/2
  Subsystem/1(Out1) -> Mux/1
  Demux/2 -> Subsystem1/1(In1)
  Demux/1 -> Subsystem/1(In1)
  u/1 -> Demux/1
  Mux/1 -> y/1

== system FourRigidBar3D/DCM(z,-3*pi//4)'1 ==
  u : Inport  PortDimensions=6
  Demux : Demux  Outputs=[3 3]
  Mux : Mux  Inputs=[3 3]
  Subsystem : Subsystem
  Subsystem1 : Subsystem
  y : Outport  VectorParamsAs1DForOutWhenUnconnected=off
  wires:
  Subsystem1/1(Out1) -> Mux/2
  Subsystem/1(Out1) -> Mux/1
  Demux/2 -> Subsystem1/1(In1)
  Demux/1 -> Subsystem/1(In1)
  u/1 -> Demux/1
  Mux/1 -> y/1

== system FourRigidBar3D/DCM(z,-3*pi//4)1 ==
  u : Inport  PortDimensions=6
  Demux : Demux  Outputs=[3 3]
  Mux : Mux  Inputs=[3 3]
  Subsystem : Subsystem
  Subsystem1 : Subsystem
  y : Outport  VectorParamsAs1DForOutWhenUnconnected=off
  wires:
  Subsystem1/1(Out1) -> Mux/2
  Subsystem/1(Out1) -> Mux/1
  Demux/2 -> Subsystem1/1(In1)
  Demux/1 -> Subsystem/1(In1)
  u/1 -> Demux/1
  Mux/1 -> y/1

== system FourRigidBar3D/DCM(z,-pi//2) ==
  u : Inport  PortDimensions=6
  Demux : Demux  Outputs=[3 3]
  Mux : Mux  Inputs=[3 3]
  Subsystem : Subsystem
  Subsystem1 : Subsystem
  y : Outport  VectorParamsAs1DForOutWhenUnconnected=off
  wires:
  Subsystem1/1(Out1) -> Mux/2
  Subsystem/1(Out1) -> Mux/1
  Demux/2 -> Subsystem1/1(In1)
  Demux/1 -> Subsystem/1(In1)
  u/1 -> Demux/1
  Mux/1 -> y/1

== system FourRigidBar3D/DCM(z,-pi//2)' ==
  u : Inport  PortDimensions=6
  Demux : Demux  Outputs=[3 3]
  Mux : Mux  Inputs=[3 3]
  Subsystem : Subsystem
  Subsystem1 : Subsystem
  y : Outport  VectorParamsAs1DForOutWhenUnconnected=off
  wires:
  Subsystem1/1(Out1) -> Mux/2
  Subsystem/1(Out1) -> Mux/1
  Demux/2 -> Subsystem1/1(In1)
  Demux/1 -> Subsystem/1(In1)
  u/1 -> Demux/1
  Mux/1 -> y/1

== system FourRigidBar3D/DCM(z,-pi//2)'1 ==
  u : Inport  PortDimensions=6
  Demux : Demux  Outputs=[3 3]
  Mux : Mux  Inputs=[3 3]
  Subsystem : Subsystem
  Subsystem1 : Subsystem
  y : Outport  VectorParamsAs1DForOutWhenUnconnected=off
  wires:
  Subsystem1/1(Out1) -> Mux/2
  Subsystem/1(Out1) -> Mux/1
  Demux/2 -> Subsystem1/1(In1)
  Demux/1 -> Subsystem/1(In1)
  u/1 -> Demux/1
  Mux/1 -> y/1

== system FourRigidBar3D/DCM(z,-pi//2)1 ==
  u : Inport  PortDimensions=6
  Demux : Demux  Outputs=[3 3]
  Mux : Mux  Inputs=[3 3]
  Subsystem : Subsystem
  Subsystem1 : Subsystem
  y : Outport  VectorParamsAs1DForOutWhenUnconnected=off
  wires:
  Subsystem1/1(Out1) -> Mux/2
  Subsystem/1(Out1) -> Mux/1
  Demux/2 -> Subsystem1/1(In1)
  Demux/1 -> Subsystem/1(In1)
  u/1 -> Demux/1
  Mux/1 -> y/1

== system FourRigidBar3D/bar # 1 ==
  Xddot,P1 : Inport  PortDimensions=6
  W_./body,P2 : Inport  Port=2  PortDimensions=6
  Demux : Demux  Outputs=[6 6]
  Gain : RCTblocks/Uncertain State Space  Tag=USS  USystem=uss(InvDyn)  UValue=[]  X0=[]  uX0=[]
  Mux : Mux  Inputs=[6 6]
  W_body/.,P1 : Outport
  Xddot,P2 : Outport  Port=2
  wires:
  Demux/2 -> Xddot,P2/1
  W_./body,P2/1 -> Mux/2
  Demux/1 -> W_body/.,P1/1
  Xddot,P1/1 -> Mux/1
  Gain/1 -> Demux/1
  Mux/1 -> Gain/1

== system FourRigidBar3D/bar # 2 ==
  Xddot,P1 : Inport  PortDimensions=6
  W_./body,P2 : Inport  Port=2  PortDimensions=6
  Demux : Demux  Outputs=[6 6]
  Gain : RCTblocks/Uncertain State Space  Tag=USS  USystem=uss(InvDyn)  UValue=[]  X0=[]  uX0=[]
  Mux : Mux  Inputs=[6 6]
  W_body/.,P1 : Outport
  Xddot,P2 : Outport  Port=2
  wires:
  Demux/2 -> Xddot,P2/1
  W_./body,P2/1 -> Mux/2
  Demux/1 -> W_body/.,P1/1
  Xddot,P1/1 -> Mux/1
  Gain/1 -> Demux/1
  Mux/1 -> Gain/1

== system FourRigidBar3D/bar # 3 ==
  Xddot,P1 : Inport  PortDimensions=6
  W_./body,P2 : Inport  Port=2  PortDimensions=6
  Demux : Demux  Outputs=[6 6]
  Gain : RCTblocks/Uncertain State Space  Tag=USS  USystem=uss(InvDyn)  UValue=[]  X0=[]  uX0=[]
  Mux : Mux  Inputs=[6 6]
  W_body/.,P1 : Outport
  Xddot,P2 : Outport  Port=2
  wires:
  Mux/1 -> Gain/1
  Gain/1 -> Demux/1
  Xddot,P1/1 -> Mux/1
  Demux/1 -> W_body/.,P1/1
  W_./body,P2/1 -> Mux/2
  Demux/2 -> Xddot,P2/1

== system FourRigidBar3D/bar# # ==
  Xddot,P1 : Inport  PortDimensions=6
  W_./body,P2 : Inport  Port=2  PortDimensions=6
  Demux : Demux  Outputs=[6 6]
  Gain : RCTblocks/Uncertain State Space  Tag=USS  USystem=uss(InvDyn)  UValue=[]  X0=[]  uX0=[]
  Mux : Mux  Inputs=[6 6]
  W_body/.,P1 : Outport
  Xddot,P2 : Outport  Port=2
  wires:
  Mux/1 -> Gain/1
  Gain/1 -> Demux/1
  Xddot,P1/1 -> Mux/1
  Demux/1 -> W_body/.,P1/1
  W_./body,P2/1 -> Mux/2
  Demux/2 -> Xddot,P2/1

== system FourRigidBar3D/loop closure constraint  ==
  xpp_C : Inport  PortDimensions=6
  xpp_P : Inport  Port=2  PortDimensions=6
  Damping Matrix : RCTblocks/Uncertain State Space  Tag=USS  USystem=ss(D_O)  UValue=[]  X0=[]  uX0=[]
  Damping Matrix1 : RCTblocks/Uncertain State Space  Tag=USS  USystem=ss(K_O)  UValue=[]  X0=[]  uX0=[]
  Integrator 1 : Integrator
  Integrator 2 : Integrator
  Kinematic model between O and C : RCTblocks/Uncertain State Space  Tag=USS  USystem=ss(TAU_OC)  UValue=[]  X0=[]  uX0=[]
  Kinematic model between O and C' : RCTblocks/Uncertain State Space  Tag=USS  USystem=ss(TAU_OC')  UValue=[]  X0=[]  uX0=[]
  Kinematic model between O and P : RCTblocks/Uncertain State Space  Tag=USS  USystem=ss(TAU_OP)  UValue=[]  X0=[]  uX0=[]
  Kinematic model between O and P' : RCTblocks/Uncertain State Space  Tag=USS  USystem=ss(TAU_OP')  UValue=[]  X0=[]  uX0=[]
  Sum : Sum  Inputs=|+-
  Sum1 : Sum  Inputs=++|
  W(./s,C) : Outport  VectorParamsAs1DForOutWhenUnconnected=off
  W(s/.,P) : Outport  Port=2  VectorParamsAs1DForOutWhenUnconnected=off
  wires:
  Kinematic model between O and C'/1 -> W(./s,C)/1
  Kinematic model between O and P'/1 -> W(s/.,P)/1
  xpp_P/1 -> Kinematic model between O and P/1
  Integrator 1/1 -> Integrator 2/1, Damping Matrix/1
  xpp_C/1 -> Kinematic model between O and C/1
  Kinematic model between O and C/1 -> Sum/1
  Sum/1 -> Integrator 1/1
  Kinematic model between O and P/1 -> Sum/2
  Damping Matrix/1 -> Sum1/2
  Damping Matrix1/1 -> Sum1/1
  Integrator 2/1 -> Damping Matrix1/1
  Sum1/1 -> Kinematic model between O and C'/1, Kinematic model between O and P'/1

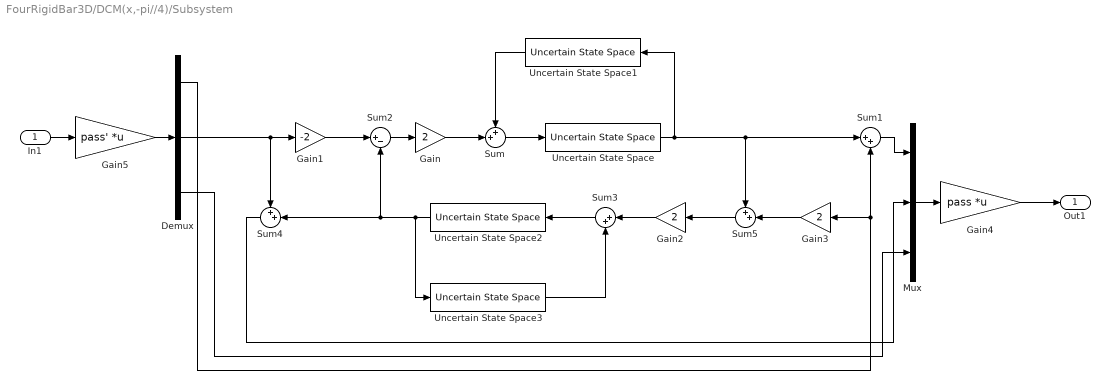
== system FourRigidBar3D/DCM(x,-pi//4)/Subsystem ==
  In1 : Inport
  Demux : Demux  Outputs=3
  Gain : Gain  Gain=2
  Gain1 : Gain  Gain=-2
  Gain2 : Gain  Gain=2
  Gain3 : Gain  Gain=2
  Gain4 : Gain  Gain=pass  Multiplication=Matrix(K*u) (u vector)
  Gain5 : Gain  Gain=pass'  Multiplication=Matrix(K*u) (u vector)
  Mux : Mux  Inputs=3
  Sum : Sum  Inputs=++|
  Sum1 : Sum  Inputs=|++
  Sum2 : Sum  Inputs=|+-
  Sum3 : Sum  Inputs=|++
  Sum4 : Sum  Inputs=++|
  Sum5 : Sum  Inputs=++|
  Uncertain State Space{,1..3} (4 alike) : RCTblocks/Uncertain State Space  Tag=USS  USystem=uss(sig4)  UValue=[]  X0=[]  uX0=[]
  Out1 : Outport  VectorParamsAs1DForOutWhenUnconnected=off
  wires:
  Gain5/1 -> Demux/1
  Gain4/1 -> Out1/1
  Uncertain State Space3/1 -> Sum3/2
  Gain2/1 -> Sum3/1
  In1/1 -> Gain5/1
  Gain/1 -> Sum/2
  Uncertain State Space2/1 -> Uncertain State Space3/1, Sum4/2, Sum2/2
  Demux/1 -> Gain3/1, Sum1/2
  Demux/3 -> Mux/3
  Mux/1 -> Gain4/1
  Sum4/1 -> Mux/2
  Sum3/1 -> Uncertain State Space2/1
  Gain1/1 -> Sum2/1
  Uncertain State Space/1 -> Uncertain State Space1/1, Sum5/1, Sum1/1
  Gain3/1 -> Sum5/2
  Sum/1 -> Uncertain State Space/1
  Demux/2 -> Sum4/1, Gain1/1
  Uncertain State Space1/1 -> Sum/1
  Sum2/1 -> Gain/1
  Sum1/1 -> Mux/1
  Sum5/1 -> Gain2/1

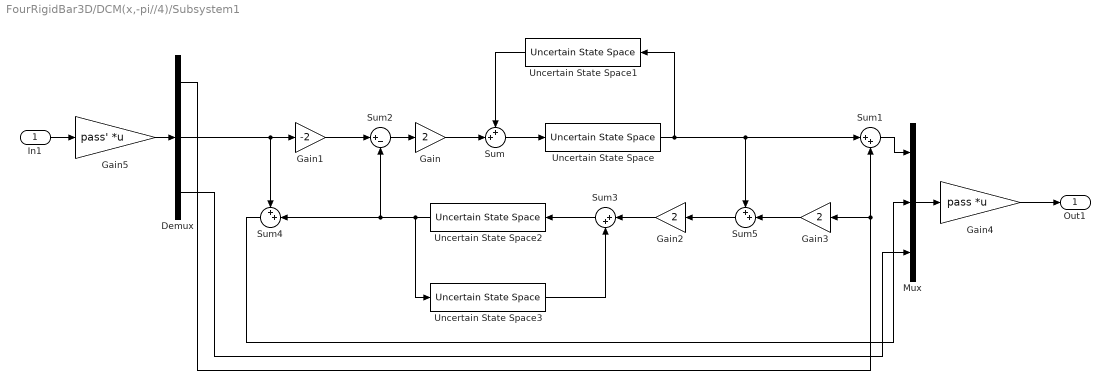
== system FourRigidBar3D/DCM(x,-pi//4)/Subsystem1 ==
  In1 : Inport
  Demux : Demux  Outputs=3
  Gain : Gain  Gain=2
  Gain1 : Gain  Gain=-2
  Gain2 : Gain  Gain=2
  Gain3 : Gain  Gain=2
  Gain4 : Gain  Gain=pass  Multiplication=Matrix(K*u) (u vector)
  Gain5 : Gain  Gain=pass'  Multiplication=Matrix(K*u) (u vector)
  Mux : Mux  Inputs=3
  Sum : Sum  Inputs=++|
  Sum1 : Sum  Inputs=|++
  Sum2 : Sum  Inputs=|+-
  Sum3 : Sum  Inputs=|++
  Sum4 : Sum  Inputs=++|
  Sum5 : Sum  Inputs=++|
  Uncertain State Space{,1..3} (4 alike) : RCTblocks/Uncertain State Space  Tag=USS  USystem=uss(sig4)  UValue=[]  X0=[]  uX0=[]
  Out1 : Outport  VectorParamsAs1DForOutWhenUnconnected=off
  wires:
  Gain5/1 -> Demux/1
  Sum5/1 -> Gain2/1
  Sum1/1 -> Mux/1
  Sum2/1 -> Gain/1
  Uncertain State Space1/1 -> Sum/1
  Demux/2 -> Gain1/1, Sum4/1
  Sum/1 -> Uncertain State Space/1
  Gain3/1 -> Sum5/2
  Uncertain State Space/1 -> Sum1/1, Sum5/1, Uncertain State Space1/1
  Gain1/1 -> Sum2/1
  Sum3/1 -> Uncertain State Space2/1
  Sum4/1 -> Mux/2
  Mux/1 -> Gain4/1
  Demux/3 -> Mux/3
  Demux/1 -> Sum1/2, Gain3/1
  Uncertain State Space2/1 -> Sum2/2, Sum4/2, Uncertain State Space3/1
  Gain/1 -> Sum/2
  In1/1 -> Gain5/1
  Gain2/1 -> Sum3/1
  Uncertain State Space3/1 -> Sum3/2
  Gain4/1 -> Out1/1

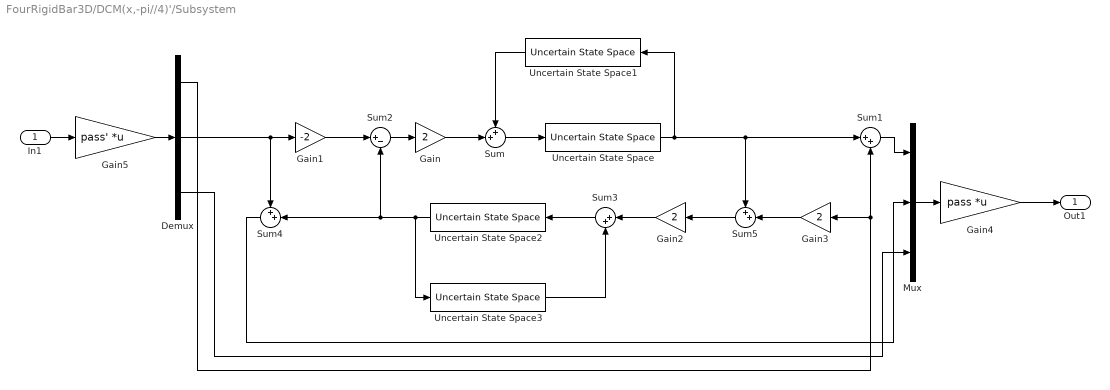
== system FourRigidBar3D/DCM(x,-pi//4)'/Subsystem ==
  In1 : Inport
  Demux : Demux  Outputs=3
  Gain : Gain  Gain=2
  Gain1 : Gain  Gain=-2
  Gain2 : Gain  Gain=2
  Gain3 : Gain  Gain=2
  Gain4 : Gain  Gain=pass  Multiplication=Matrix(K*u) (u vector)
  Gain5 : Gain  Gain=pass'  Multiplication=Matrix(K*u) (u vector)
  Mux : Mux  Inputs=3
  Sum : Sum  Inputs=++|
  Sum1 : Sum  Inputs=|++
  Sum2 : Sum  Inputs=|+-
  Sum3 : Sum  Inputs=|++
  Sum4 : Sum  Inputs=++|
  Sum5 : Sum  Inputs=++|
  Uncertain State Space{,1..3} (4 alike) : RCTblocks/Uncertain State Space  Tag=USS  USystem=uss(sig4)  UValue=[]  X0=[]  uX0=[]
  Out1 : Outport  VectorParamsAs1DForOutWhenUnconnected=off
  wires:
  Gain5/1 -> Demux/1
  Gain4/1 -> Out1/1
  Uncertain State Space3/1 -> Sum3/2
  Gain2/1 -> Sum3/1
  In1/1 -> Gain5/1
  Gain/1 -> Sum/2
  Uncertain State Space2/1 -> Uncertain State Space3/1, Sum4/2, Sum2/2
  Demux/1 -> Gain3/1, Sum1/2
  Demux/3 -> Mux/3
  Mux/1 -> Gain4/1
  Sum4/1 -> Mux/2
  Sum3/1 -> Uncertain State Space2/1
  Gain1/1 -> Sum2/1
  Uncertain State Space/1 -> Uncertain State Space1/1, Sum5/1, Sum1/1
  Gain3/1 -> Sum5/2
  Sum/1 -> Uncertain State Space/1
  Demux/2 -> Sum4/1, Gain1/1
  Uncertain State Space1/1 -> Sum/1
  Sum2/1 -> Gain/1
  Sum1/1 -> Mux/1
  Sum5/1 -> Gain2/1

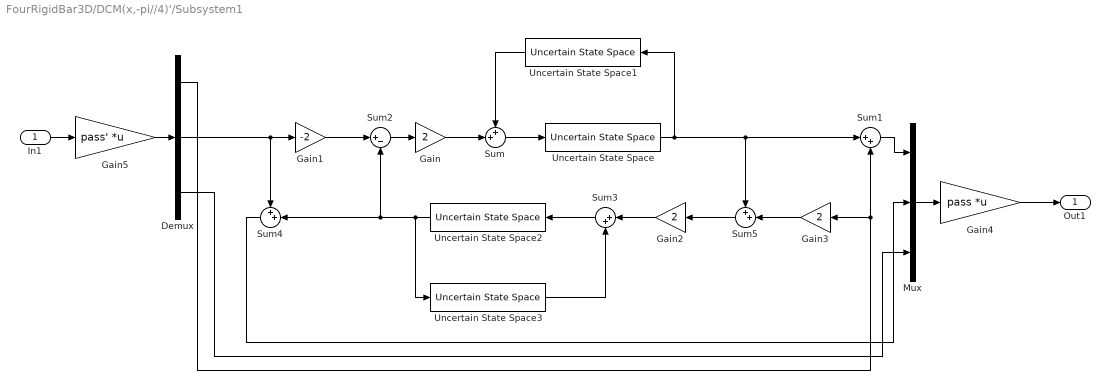
== system FourRigidBar3D/DCM(x,-pi//4)'/Subsystem1 ==
  In1 : Inport
  Demux : Demux  Outputs=3
  Gain : Gain  Gain=2
  Gain1 : Gain  Gain=-2
  Gain2 : Gain  Gain=2
  Gain3 : Gain  Gain=2
  Gain4 : Gain  Gain=pass  Multiplication=Matrix(K*u) (u vector)
  Gain5 : Gain  Gain=pass'  Multiplication=Matrix(K*u) (u vector)
  Mux : Mux  Inputs=3
  Sum : Sum  Inputs=++|
  Sum1 : Sum  Inputs=|++
  Sum2 : Sum  Inputs=|+-
  Sum3 : Sum  Inputs=|++
  Sum4 : Sum  Inputs=++|
  Sum5 : Sum  Inputs=++|
  Uncertain State Space{,1..3} (4 alike) : RCTblocks/Uncertain State Space  Tag=USS  USystem=uss(sig4)  UValue=[]  X0=[]  uX0=[]
  Out1 : Outport  VectorParamsAs1DForOutWhenUnconnected=off
  wires:
  Gain5/1 -> Demux/1
  Sum5/1 -> Gain2/1
  Sum1/1 -> Mux/1
  Sum2/1 -> Gain/1
  Uncertain State Space1/1 -> Sum/1
  Demux/2 -> Gain1/1, Sum4/1
  Sum/1 -> Uncertain State Space/1
  Gain3/1 -> Sum5/2
  Uncertain State Space/1 -> Sum1/1, Sum5/1, Uncertain State Space1/1
  Gain1/1 -> Sum2/1
  Sum3/1 -> Uncertain State Space2/1
  Sum4/1 -> Mux/2
  Mux/1 -> Gain4/1
  Demux/3 -> Mux/3
  Demux/1 -> Sum1/2, Gain3/1
  Uncertain State Space2/1 -> Sum2/2, Sum4/2, Uncertain State Space3/1
  Gain/1 -> Sum/2
  In1/1 -> Gain5/1
  Gain2/1 -> Sum3/1
  Uncertain State Space3/1 -> Sum3/2
  Gain4/1 -> Out1/1

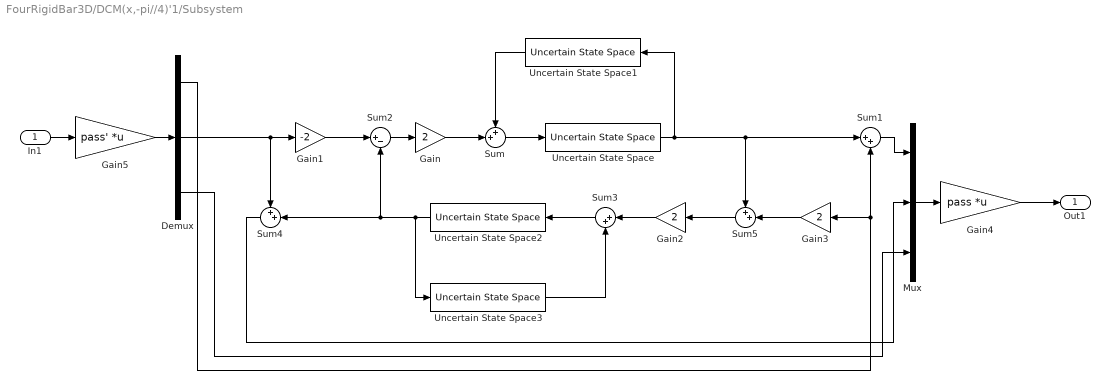
== system FourRigidBar3D/DCM(x,-pi//4)'1/Subsystem ==
  In1 : Inport
  Demux : Demux  Outputs=3
  Gain : Gain  Gain=2
  Gain1 : Gain  Gain=-2
  Gain2 : Gain  Gain=2
  Gain3 : Gain  Gain=2
  Gain4 : Gain  Gain=pass  Multiplication=Matrix(K*u) (u vector)
  Gain5 : Gain  Gain=pass'  Multiplication=Matrix(K*u) (u vector)
  Mux : Mux  Inputs=3
  Sum : Sum  Inputs=++|
  Sum1 : Sum  Inputs=|++
  Sum2 : Sum  Inputs=|+-
  Sum3 : Sum  Inputs=|++
  Sum4 : Sum  Inputs=++|
  Sum5 : Sum  Inputs=++|
  Uncertain State Space{,1..3} (4 alike) : RCTblocks/Uncertain State Space  Tag=USS  USystem=uss(sig4)  UValue=[]  X0=[]  uX0=[]
  Out1 : Outport  VectorParamsAs1DForOutWhenUnconnected=off
  wires:
  Gain5/1 -> Demux/1
  Gain4/1 -> Out1/1
  Uncertain State Space3/1 -> Sum3/2
  Gain2/1 -> Sum3/1
  In1/1 -> Gain5/1
  Gain/1 -> Sum/2
  Uncertain State Space2/1 -> Uncertain State Space3/1, Sum4/2, Sum2/2
  Demux/1 -> Gain3/1, Sum1/2
  Demux/3 -> Mux/3
  Mux/1 -> Gain4/1
  Sum4/1 -> Mux/2
  Sum3/1 -> Uncertain State Space2/1
  Gain1/1 -> Sum2/1
  Uncertain State Space/1 -> Uncertain State Space1/1, Sum5/1, Sum1/1
  Gain3/1 -> Sum5/2
  Sum/1 -> Uncertain State Space/1
  Demux/2 -> Sum4/1, Gain1/1
  Uncertain State Space1/1 -> Sum/1
  Sum2/1 -> Gain/1
  Sum1/1 -> Mux/1
  Sum5/1 -> Gain2/1

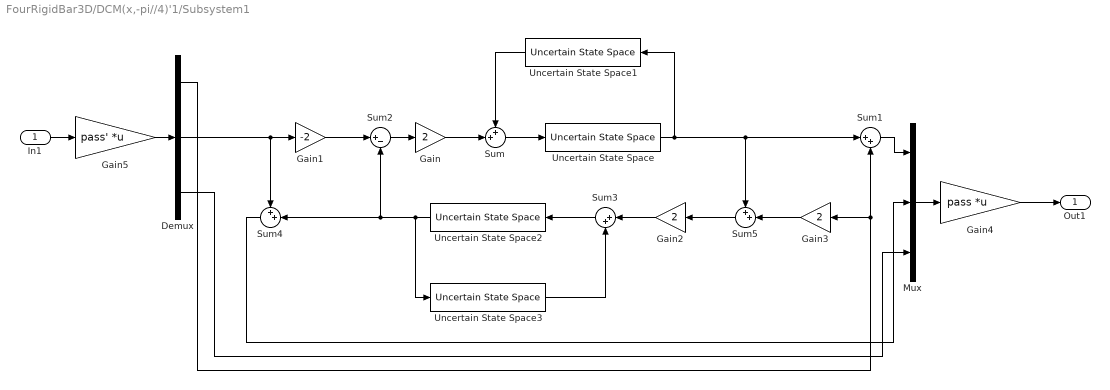
== system FourRigidBar3D/DCM(x,-pi//4)'1/Subsystem1 ==
  In1 : Inport
  Demux : Demux  Outputs=3
  Gain : Gain  Gain=2
  Gain1 : Gain  Gain=-2
  Gain2 : Gain  Gain=2
  Gain3 : Gain  Gain=2
  Gain4 : Gain  Gain=pass  Multiplication=Matrix(K*u) (u vector)
  Gain5 : Gain  Gain=pass'  Multiplication=Matrix(K*u) (u vector)
  Mux : Mux  Inputs=3
  Sum : Sum  Inputs=++|
  Sum1 : Sum  Inputs=|++
  Sum2 : Sum  Inputs=|+-
  Sum3 : Sum  Inputs=|++
  Sum4 : Sum  Inputs=++|
  Sum5 : Sum  Inputs=++|
  Uncertain State Space{,1..3} (4 alike) : RCTblocks/Uncertain State Space  Tag=USS  USystem=uss(sig4)  UValue=[]  X0=[]  uX0=[]
  Out1 : Outport  VectorParamsAs1DForOutWhenUnconnected=off
  wires:
  Gain5/1 -> Demux/1
  Sum5/1 -> Gain2/1
  Sum1/1 -> Mux/1
  Sum2/1 -> Gain/1
  Uncertain State Space1/1 -> Sum/1
  Demux/2 -> Gain1/1, Sum4/1
  Sum/1 -> Uncertain State Space/1
  Gain3/1 -> Sum5/2
  Uncertain State Space/1 -> Sum1/1, Sum5/1, Uncertain State Space1/1
  Gain1/1 -> Sum2/1
  Sum3/1 -> Uncertain State Space2/1
  Sum4/1 -> Mux/2
  Mux/1 -> Gain4/1
  Demux/3 -> Mux/3
  Demux/1 -> Sum1/2, Gain3/1
  Uncertain State Space2/1 -> Sum2/2, Sum4/2, Uncertain State Space3/1
  Gain/1 -> Sum/2
  In1/1 -> Gain5/1
  Gain2/1 -> Sum3/1
  Uncertain State Space3/1 -> Sum3/2
  Gain4/1 -> Out1/1

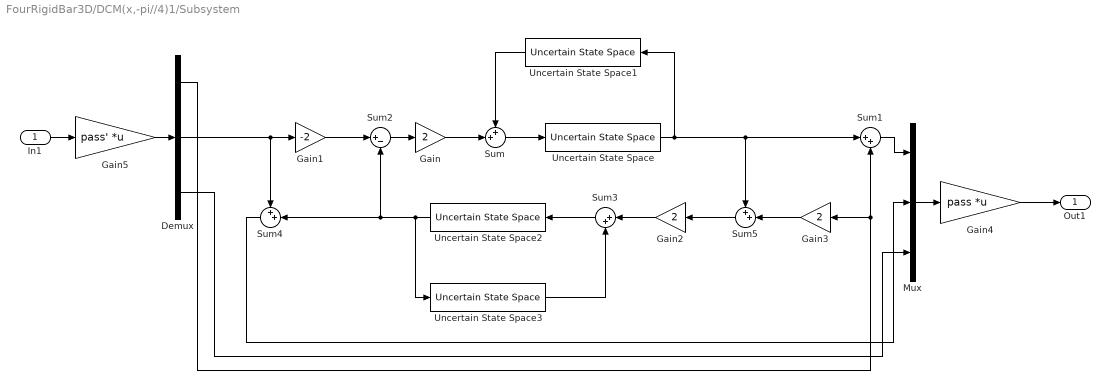
== system FourRigidBar3D/DCM(x,-pi//4)1/Subsystem ==
  In1 : Inport
  Demux : Demux  Outputs=3
  Gain : Gain  Gain=2
  Gain1 : Gain  Gain=-2
  Gain2 : Gain  Gain=2
  Gain3 : Gain  Gain=2
  Gain4 : Gain  Gain=pass  Multiplication=Matrix(K*u) (u vector)
  Gain5 : Gain  Gain=pass'  Multiplication=Matrix(K*u) (u vector)
  Mux : Mux  Inputs=3
  Sum : Sum  Inputs=++|
  Sum1 : Sum  Inputs=|++
  Sum2 : Sum  Inputs=|+-
  Sum3 : Sum  Inputs=|++
  Sum4 : Sum  Inputs=++|
  Sum5 : Sum  Inputs=++|
  Uncertain State Space{,1..3} (4 alike) : RCTblocks/Uncertain State Space  Tag=USS  USystem=uss(sig4)  UValue=[]  X0=[]  uX0=[]
  Out1 : Outport  VectorParamsAs1DForOutWhenUnconnected=off
  wires:
  Gain5/1 -> Demux/1
  Gain4/1 -> Out1/1
  Uncertain State Space3/1 -> Sum3/2
  Gain2/1 -> Sum3/1
  In1/1 -> Gain5/1
  Gain/1 -> Sum/2
  Uncertain State Space2/1 -> Uncertain State Space3/1, Sum4/2, Sum2/2
  Demux/1 -> Gain3/1, Sum1/2
  Demux/3 -> Mux/3
  Mux/1 -> Gain4/1
  Sum4/1 -> Mux/2
  Sum3/1 -> Uncertain State Space2/1
  Gain1/1 -> Sum2/1
  Uncertain State Space/1 -> Uncertain State Space1/1, Sum5/1, Sum1/1
  Gain3/1 -> Sum5/2
  Sum/1 -> Uncertain State Space/1
  Demux/2 -> Sum4/1, Gain1/1
  Uncertain State Space1/1 -> Sum/1
  Sum2/1 -> Gain/1
  Sum1/1 -> Mux/1
  Sum5/1 -> Gain2/1

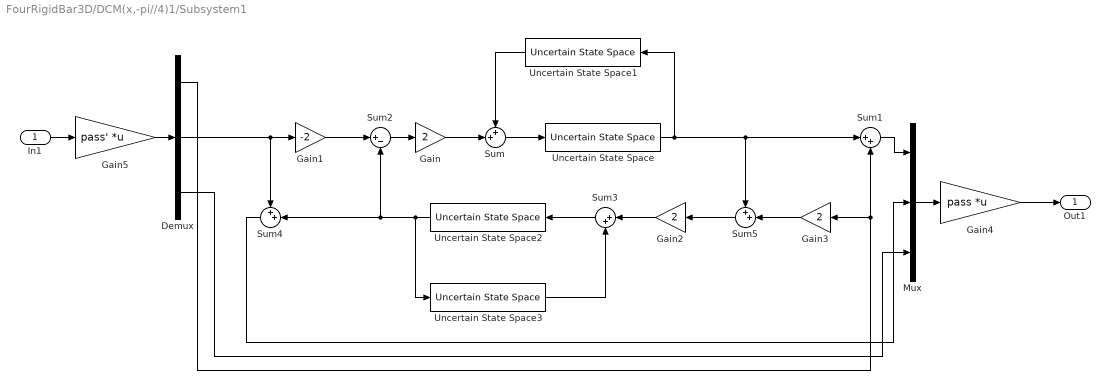
== system FourRigidBar3D/DCM(x,-pi//4)1/Subsystem1 ==
  In1 : Inport
  Demux : Demux  Outputs=3
  Gain : Gain  Gain=2
  Gain1 : Gain  Gain=-2
  Gain2 : Gain  Gain=2
  Gain3 : Gain  Gain=2
  Gain4 : Gain  Gain=pass  Multiplication=Matrix(K*u) (u vector)
  Gain5 : Gain  Gain=pass'  Multiplication=Matrix(K*u) (u vector)
  Mux : Mux  Inputs=3
  Sum : Sum  Inputs=++|
  Sum1 : Sum  Inputs=|++
  Sum2 : Sum  Inputs=|+-
  Sum3 : Sum  Inputs=|++
  Sum4 : Sum  Inputs=++|
  Sum5 : Sum  Inputs=++|
  Uncertain State Space{,1..3} (4 alike) : RCTblocks/Uncertain State Space  Tag=USS  USystem=uss(sig4)  UValue=[]  X0=[]  uX0=[]
  Out1 : Outport  VectorParamsAs1DForOutWhenUnconnected=off
  wires:
  Gain5/1 -> Demux/1
  Sum5/1 -> Gain2/1
  Sum1/1 -> Mux/1
  Sum2/1 -> Gain/1
  Uncertain State Space1/1 -> Sum/1
  Demux/2 -> Gain1/1, Sum4/1
  Sum/1 -> Uncertain State Space/1
  Gain3/1 -> Sum5/2
  Uncertain State Space/1 -> Sum1/1, Sum5/1, Uncertain State Space1/1
  Gain1/1 -> Sum2/1
  Sum3/1 -> Uncertain State Space2/1
  Sum4/1 -> Mux/2
  Mux/1 -> Gain4/1
  Demux/3 -> Mux/3
  Demux/1 -> Sum1/2, Gain3/1
  Uncertain State Space2/1 -> Sum2/2, Sum4/2, Uncertain State Space3/1
  Gain/1 -> Sum/2
  In1/1 -> Gain5/1
  Gain2/1 -> Sum3/1
  Uncertain State Space3/1 -> Sum3/2
  Gain4/1 -> Out1/1

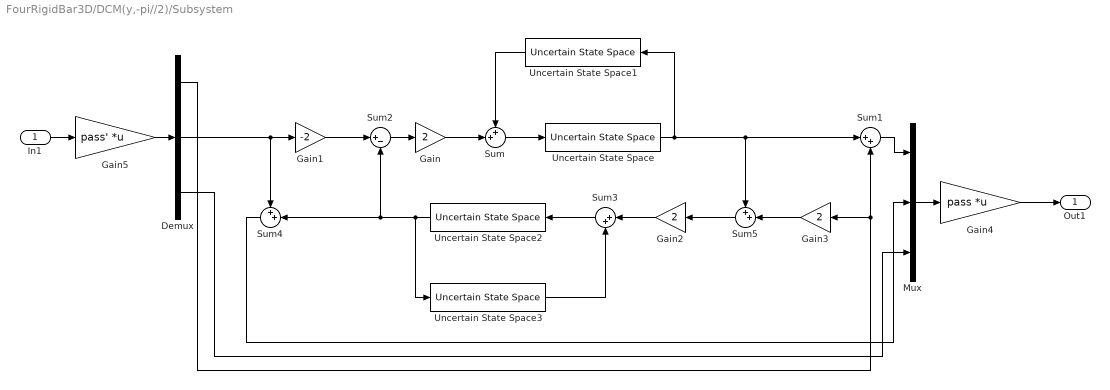
== system FourRigidBar3D/DCM(y,-pi//2)/Subsystem ==
  In1 : Inport
  Demux : Demux  Outputs=3
  Gain : Gain  Gain=2
  Gain1 : Gain  Gain=-2
  Gain2 : Gain  Gain=2
  Gain3 : Gain  Gain=2
  Gain4 : Gain  Gain=pass  Multiplication=Matrix(K*u) (u vector)
  Gain5 : Gain  Gain=pass'  Multiplication=Matrix(K*u) (u vector)
  Mux : Mux  Inputs=3
  Sum : Sum  Inputs=++|
  Sum1 : Sum  Inputs=|++
  Sum2 : Sum  Inputs=|+-
  Sum3 : Sum  Inputs=|++
  Sum4 : Sum  Inputs=++|
  Sum5 : Sum  Inputs=++|
  Uncertain State Space{,1..3} (4 alike) : RCTblocks/Uncertain State Space  Tag=USS  USystem=uss(sig4)  UValue=[]  X0=[]  uX0=[]
  Out1 : Outport  VectorParamsAs1DForOutWhenUnconnected=off
  wires:
  Gain5/1 -> Demux/1
  Gain4/1 -> Out1/1
  Uncertain State Space3/1 -> Sum3/2
  Gain2/1 -> Sum3/1
  In1/1 -> Gain5/1
  Gain/1 -> Sum/2
  Uncertain State Space2/1 -> Uncertain State Space3/1, Sum4/2, Sum2/2
  Demux/1 -> Gain3/1, Sum1/2
  Demux/3 -> Mux/3
  Mux/1 -> Gain4/1
  Sum4/1 -> Mux/2
  Sum3/1 -> Uncertain State Space2/1
  Gain1/1 -> Sum2/1
  Uncertain State Space/1 -> Uncertain State Space1/1, Sum5/1, Sum1/1
  Gain3/1 -> Sum5/2
  Sum/1 -> Uncertain State Space/1
  Demux/2 -> Sum4/1, Gain1/1
  Uncertain State Space1/1 -> Sum/1
  Sum2/1 -> Gain/1
  Sum1/1 -> Mux/1
  Sum5/1 -> Gain2/1
